simulink model "Resistive_Model_1_v2"  (R2020a)
settings: Solver=VariableStepAuto  StartTime=0.0  StopTime=10.0  RelTol=1e-3
libraries: powerlib x3, re_lib x1
settings Model: Creator=mitch  LastModifiedBy=mitch

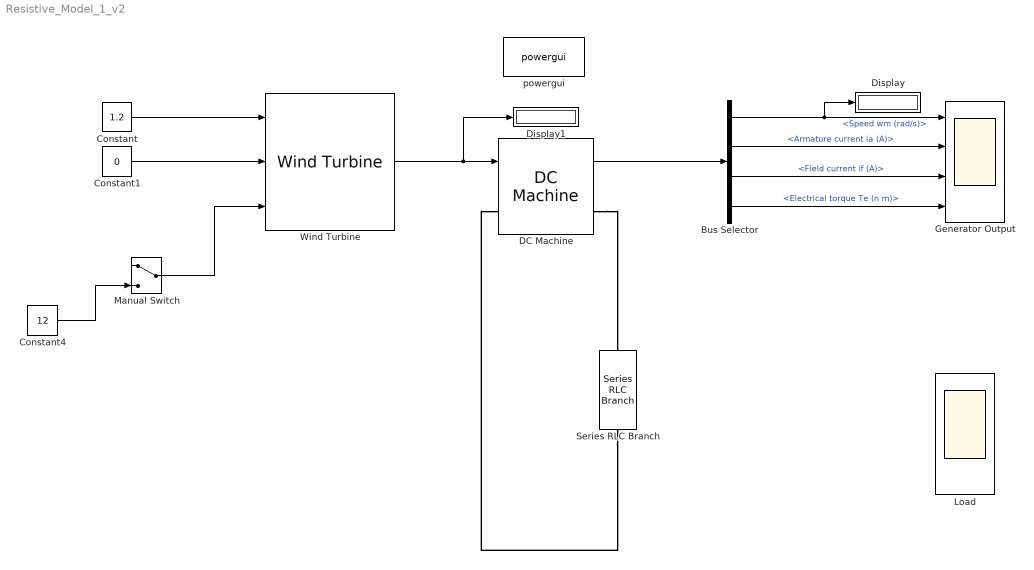
== system Resistive_Model_1_v2 ==
  Bus Selector : BusSelector  OutputSignals=Speed wm (rad/s),Armature current ia (A),Field current if (A),Electrical torque Te (n m)
  Constant : Constant  Value=1.2
  Constant1 : Constant  Value=0
  Constant4 : Constant  Value=12
  DC Machine : powerlib/Machines/DC Machine  PresetModel=No  MechanicalLoad=Torque TL  FieldType=Permanent magnet  ShowDetailedParameters=on  MeasurementBus=off  RLa="[ 0.6  0.012]"  RLf="[ 240  120]"  Laf=1.8  MachineConstant=Torque constant (N.m/A)  Ke=1.8  Kt=1.8  J=1  Bm=0  Tf=0  w0=1  Ifinit=1  TsPowergui=0  TsBlock=-1
  Display : Display
  Display1 : Display
  Generator Output : Scope  NumInputPorts=4
  Load : Scope  NumInputPorts=3
  Manual Switch : ManualSwitch
  Series RLC Branch : powerlib/Elements/Series RLC Branch  LConnTagsString=__new0  RConnTagsString=__new0  BranchType=R  Resistance=1  Inductance=1e-3  SetiL0=off  InitialCurrent=0  Capacitance=1e-6  Setx0=off  InitialVoltage=0  Measurements=None
  Wind Turbine : re_lib/Wind Generation/Wind Turbine  Pnom=460  Pelec_base=460/0.9  wind_base=8  P_wind_base=0.73  speed_nom=1.2  pitch_angle=0  c1_c6="[0.51763          116          0.4            5           21     0.006795]"  cp_nom=0.48  lambda_nom=8.1
      settings: SourceProductBaseCode=PS
  powergui : powerlib/powergui  Priority=1  SimulationMode=Continuous  SampleTime=50e-6  frequency=60  Iterations=50  frequencyindice=60  Pbase=100e6  ErrMax=1e-4  UnitsV=kV  UnitsW=MW  buscounter=0  FunctionMessages=off  echomessages=off  EnableUseOfTLC=off  CurrentSourceSwitches=off  DisableSnubberDevices=off  DisableRonSwitches=off  DisableVfSwitches=off  DisplayEquations=off  AutomaticDiscreteSolvers=off  SolverType=Tustin/Backward Euler (TBE)  Interpol=off  ExternalGateDelay=off  methode=off  Ts=100  x0status=blocks  SPID=on  SwTol=0  HookPort=off  NonlinearTolerance=1e-4  nMaxIteration=100  ContinueOnMaxIteration=off  RestoreLinks=warning  ResistiveCurrentMeasurement=off  Frange=[0:2:500]  Ylog=off  Xlog=on  ShowGrid=off  save=off  variable=ZData  structure=0  ZoomFFT=off  StartTime=0.0  cycles=1  DisplayStyle=1  fundamental=60  FreqAxis=off  MaxFrequency=1000  frequencyindicesteady=1  RmsSteady=1  display=off
  wires:
  Wind Turbine/1 -> Display1/1, DC Machine/1
  Constant1/1 -> Wind Turbine/2
  Constant/1 -> Wind Turbine/1
  Manual Switch/1 -> Wind Turbine/3
  Constant4/1 -> Manual Switch/2
  ? -> Manual Switch/1
  DC Machine/1 -> Bus Selector/1
  Bus Selector/1 -> Display/1, Generator Output/1  "<Speed wm (rad/s)>"
  Bus Selector/2 -> Generator Output/2  "<Armature current ia (A)>"
  Bus Selector/3 -> Generator Output/3  "<Field current if (A)>"
  Bus Selector/4 -> Generator Output/4  "<Electrical torque Te (n m)>"
  connections:
  DC Machine/RConn1 -- Series RLC Branch/LConn1
  Series RLC Branch/RConn1 -- DC Machine/LConn1
